simulink model "AMK_model_testSimulation"  (R2022b)
settings: Solver=FixedStepAuto  StartTime=0.0  StopTime=40  FixedStep=1e-2  RelTol=1e-3
libraries: AMK_model_lib x1
settings Model: Creator=dr_pa  LastModifiedBy=dr_pa
settings DataIOCC: ExternalInput=AMK_physicsModel_test.getElement('TargetVelocity_R'),AMK_physicsModel_test.getElement('TorqueLimPos_R'),AMK_physicsModel_test.getElement('TorqueLimNeg_R'),AMK_physicsModel_test.getElement('Mot_running'),AMK_physicsModel_test.getElement('p_brakePedalPos'),AMK_physicsModel_test.getElement('TargetVelocity_L'),AMK_physicsModel_test.getElement('TorqueLimPos_L'),AMK_physicsModel_test.getElement('TorqueLimNeg_L')  LoadExternalInput=on

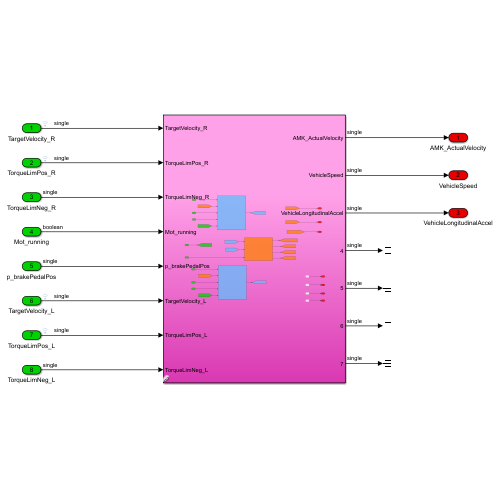
[thumbnail: Simulink's stored preview of the top-level diagram]
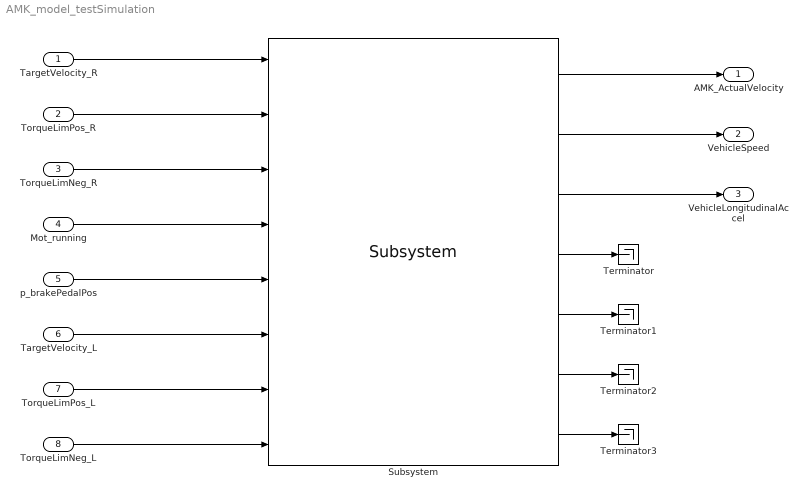
== system AMK_model_testSimulation ==
  TargetVelocity_R : Inport
  TorqueLimPos_R : Inport  Port=2
  TorqueLimNeg_R : Inport  Port=3
  Mot_running : Inport  Port=4
  p_brakePedalPos : Inport  Port=5  OutDataTypeStr=single
  TargetVelocity_L : Inport  Port=6
  TorqueLimPos_L : Inport  Port=7
  TorqueLimNeg_L : Inport  Port=8
  Subsystem : AMK_model_lib/AMK_PLANT/Subsystem  SystemSampleTime=-1  VariantActivationTime=update diagram  Latency=0  AutoFrameSizeCalculation=off
  Terminator{,1..3} (4 alike) : Terminator
  AMK_ActualVelocity : Outport
  VehicleSpeed : Outport  Port=2
  VehicleLongitudinalAccel : Outport  Port=3
  wires:
  Subsystem/2 -> VehicleSpeed/1
  Subsystem/1 -> AMK_ActualVelocity/1
  Subsystem/3 -> VehicleLongitudinalAccel/1
  Mot_running/1 -> Subsystem/4
  TorqueLimNeg_L/1 -> Subsystem/8
  TargetVelocity_R/1 -> Subsystem/1
  TorqueLimPos_R/1 -> Subsystem/2
  TorqueLimNeg_R/1 -> Subsystem/3
  p_brakePedalPos/1 -> Subsystem/5
  TargetVelocity_L/1 -> Subsystem/6
  TorqueLimPos_L/1 -> Subsystem/7
  Subsystem/4 -> Terminator/1
  Subsystem/5 -> Terminator1/1
  Subsystem/6 -> Terminator2/1
  Subsystem/7 -> Terminator3/1
